simulink model "gm_uz_ssi_interface_2023a"  (R2023a)
settings: Solver=FixedStepDiscrete  StartTime=0.0  StopTime=0.0025  RelTol=1e-3
undefined symbols (not defined in the file or in its folder): binary_or_gray, bit_sum, delay_first_clk_on_off, f_ADC, f_clock, PLL, ssi_clk_divider, ssi_encoder_bit_width_multi_turn, ssi_encoder_bit_width_single_turn, ssi_encoder_number_of_status_bits, t_ADC, t_clock
libraries: hdlmdlgenlib x111, hdlsllib x62, simulink x27, simulink_extras x7
(part 1 of 4)
settings Model: Creator=micha  LastModifiedBy=micha
settings SolverCC: AlgebraicLoopSolver=TrustRegion
settings DataIOCC: LimitDataPoints=on  SaveOutput=off  SaveTime=off
settings OptimizationCC: BlockReduction=off  ConditionallyExecuteInputs=off  DefaultParameterBehavior=Inlined  LifeSpan=inf
settings DebuggingCC: AlgebraicLoopMsg=error  ArtificialAlgebraicLoopMsg=none  InheritedTsInSrcMsg=none  SingleTaskRateTransMsg=error  UnconnectedInputMsg=warning  UnconnectedOutputMsg=warning  UnconnectedLineMsg=warning  AllowSymbolicDim=off  StrictBusMsg=ErrorOnBusTreatedAsVector  SFUnexpectedBacktrackingDiag=warning  SFNoUnconditionalDefaultTransitionDiag=warning  SFExecutionAtInitializationDiag=none  ArithmeticOperatorsInVariantConditions=warning
settings HardwareCC: ProdBitPerPointer=32  ProdBitPerSizeT=32  ProdBitPerPtrDiffT=32  ProdLargestAtomicFloat=None  ProdIntDivRoundTo=Undefined  ProdEndianess=Unspecified  ProdWordSize=32  ProdHWDeviceType=ASIC/FPGA->ASIC/FPGA  ProdEqTarget=off
settings ModelReferenceCC: EnableRefExpFcnMdlSchedulingChecks=on
settings SFSimCC: SimUseLocalCustomCode=off  CustomCodeUndefinedFunction=UseInterfaceOnly
settings RTWCC: RTWUseLocalCustomCode=off  DLArmComputeVersion=19.05
settings CodeAppCC: StateflowObjectComments=on
settings GRTTargetCC: TargetLangStandard=C89/C90 (ANSI)
settings ConfigComp: CovScope=ReferencedModels  CovMetricSettings=dw  CovSaveCumulativeToWorkspaceVar=on  CovSaveSingleToWorkspaceVar=on  CovExternalEMLEnable=off  CovSFcnEnable=off

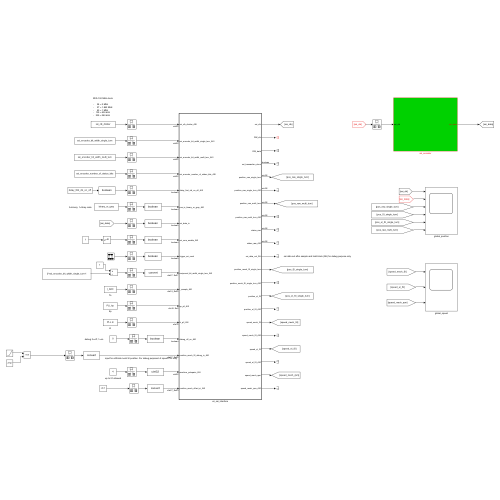
[thumbnail: Simulink's stored preview of the top-level diagram]
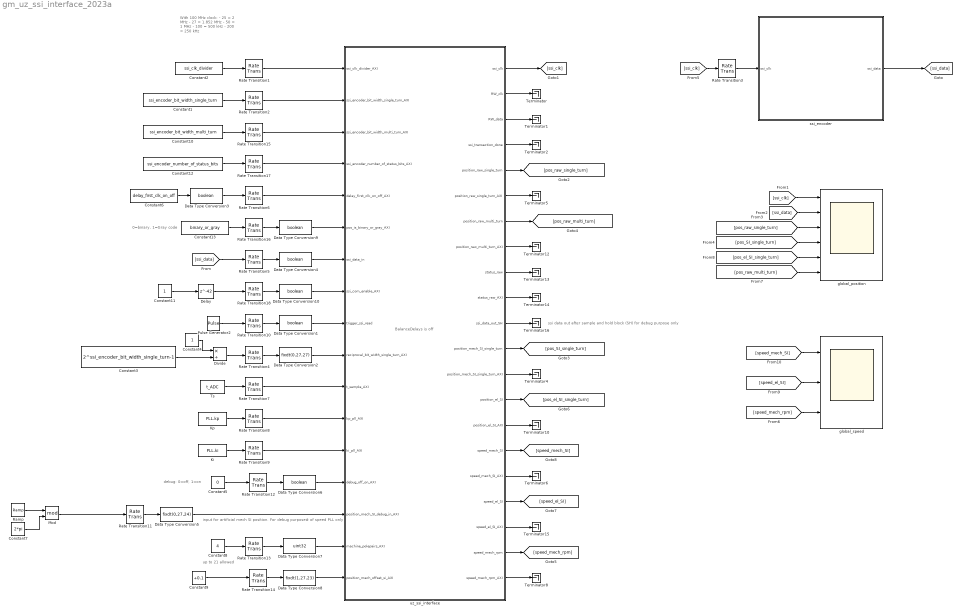
== system gm_uz_ssi_interface_2023a ==
  note: 0=binary, 1=Gray code
  note: With 100 MHz clock:
      |
      | -     25 = 2 MHz
      | -     27 = 1.852 MHz
      | -     50 = 1 MHz
      | -   100 = 500 kHz
      | -   200 = 250 kHz
  note: BalanceDelays is off
  note: debug: 0=off, 1=on
  note: up to 21 allowed
  note: ssi data out after sample and hold block (SH) for debug purpose only
  note: input for artificial mech SI position. For debug purpose# of speed PLL only
  Constant1 : Constant  Value=ssi_encoder_bit_width_single_turn  OutDataTypeStr=uint32  SampleTime=t_clock
  Constant10 : Constant  Value=ssi_encoder_bit_width_multi_turn  OutDataTypeStr=uint32  SampleTime=t_clock
  Constant11 : Constant  SampleTime=t_clock
  Constant12 : Constant  Value=ssi_encoder_number_of_status_bits  OutDataTypeStr=uint32  SampleTime=t_clock
  Constant13 : Constant  Value=binary_or_gray  OutDataTypeStr=uint32  SampleTime=t_clock
  Constant2 : Constant  Value=ssi_clk_divider  OutDataTypeStr=uint32  SampleTime=t_clock
  Constant3 : Constant  Value=2^ssi_encoder_bit_width_single_turn-1  OutDataTypeStr=double  SampleTime=t_clock
  Constant4 : Constant  SampleTime=t_clock
  Constant5 : Constant  Value=0  SampleTime=t_clock
  Constant6 : Constant  Value=delay_first_clk_on_off  OutDataTypeStr=uint32  SampleTime=t_clock
  Constant7 : Constant  Value=2*pi  SampleTime=t_clock
  Constant8 : Constant  Value=4  SampleTime=t_clock
  Constant9 : Constant  Value=+0.1  SampleTime=t_clock
  Data Type Conversion{1,3..4,6,9..10} (6 alike) : DataTypeConversion  OutDataTypeStr=boolean  SaturateOnIntegerOverflow=off  RndMeth=Floor
  Data Type Conversion2 : DataTypeConversion  OutDataTypeStr=fixdt(0,27,27)  SaturateOnIntegerOverflow=off  RndMeth=Floor
  Data Type Conversion5 : DataTypeConversion  OutDataTypeStr=fixdt(0,27,24)  SaturateOnIntegerOverflow=off  RndMeth=Floor
  Data Type Conversion7 : DataTypeConversion  OutDataTypeStr=uint32  SaturateOnIntegerOverflow=off  RndMeth=Floor
  Data Type Conversion8 : DataTypeConversion  OutDataTypeStr=fixdt(1,27,23)  SaturateOnIntegerOverflow=off  RndMeth=Floor
  Delay : Delay  DelayLength=42
  Divide : Product  Inputs=*/
  Ki : Constant  Value=PLL.ki  OutDataTypeStr=fixdt(0,18,0)  SampleTime=-1
  Kp : Constant  Value=PLL.kp  OutDataTypeStr=fixdt(0,18,5)  SampleTime=-1
  Mod : Math  Operator=mod
  Pulse Generator2 : DiscretePulseGenerator  Period=f_clock/f_ADC  PulseWidth=0.04*f_clock/f_ADC  PhaseDelay=250  SampleTime=t_clock
  Ramp : simulink/Sources/Ramp  slope=2*pi*100  start=7.5e-5  InitialOutput=0
  Rate Transition{1..18} (18 alike) : RateTransition  OutPortSampleTime=t_clock
  Terminator{,1..2,4..6,8,10,12..16} (13 alike) : Terminator
  Ts : Constant  Value=t_ADC  OutDataTypeStr=fixdt(0,18,24)  SampleTime=-1
  global_position : Scope  NumInputPorts=6
  global_speed : Scope  NumInputPorts=3
  ssi_encoder : Subsystem
  uz_ssi_interface : Subsystem  TreatAsAtomicUnit=on
  wires:
  [speed_el_SI] -> global_speed/2
  [speed_mech_SI] -> global_speed/1
  [pos_el_SI_single_turn] -> global_position/5
  [pos_raw_multi_turn] -> global_position/6
  [speed_mech_rpm] -> global_speed/3
  [ssi_clk] -> Rate Transition3/1
  Delay/1 -> Rate Transition18/1
  uz_ssi_interface/20(speed_mech_rpm) -> [speed_mech_rpm]
  uz_ssi_interface/11(ssi_data_out_SH) -> Terminator16/1
  uz_ssi_interface/12(position_mech_SI_single_turn) -> [pos_SI_single_turn]
  [pos_SI_single_turn] -> global_position/4
  [pos_raw_single_turn] -> global_position/3
  uz_ssi_interface/5(position_raw_single_turn) -> [pos_raw_single_turn]
  [ssi_data] -> global_position/2
  [ssi_clk] -> global_position/1
  uz_ssi_interface/18(speed_el_SI) -> [speed_el_SI]
  uz_ssi_interface/19(speed_el_SI_AXI) -> Terminator15/1
  uz_ssi_interface/10(status_raw_AXI) -> Terminator14/1
  uz_ssi_interface/9(status_raw) -> Terminator13/1
  uz_ssi_interface/8(position_raw_multi_turn_AXI) -> Terminator12/1
  uz_ssi_interface/7(position_raw_multi_turn) -> [pos_raw_multi_turn]
  Constant11/1 -> Delay/1
  Rate Transition18/1 -> Data Type Conversion10/1
  Data Type Conversion10/1 -> uz_ssi_interface/8(ssi_com_enable_AXI)
  Constant12/1 -> Rate Transition17/1
  Rate Transition17/1 -> uz_ssi_interface/4(ssi_encoder_number_of_status_bits_AXI)
  Data Type Conversion9/1 -> uz_ssi_interface/6(pos_is_binary_or_gray_AXI)
  Constant13/1 -> Rate Transition16/1
  Rate Transition16/1 -> Data Type Conversion9/1
  Constant10/1 -> Rate Transition15/1
  Rate Transition15/1 -> uz_ssi_interface/3(ssi_encoder_bit_width_multi_turn_AXI)
  uz_ssi_interface/15(position_el_SI_AXI) -> Terminator10/1
  uz_ssi_interface/14(position_el_SI) -> [pos_el_SI_single_turn]
  Data Type Conversion8/1 -> uz_ssi_interface/17(position_mech_offset_si_AXI)
  Constant9/1 -> Rate Transition14/1
  Rate Transition14/1 -> Data Type Conversion8/1
  Constant8/1 -> Rate Transition13/1
  Data Type Conversion7/1 -> uz_ssi_interface/16(machine_polepairs_AXI)
  Rate Transition13/1 -> Data Type Conversion7/1
  uz_ssi_interface/21(speed_mech_rpm_AXI) -> Terminator8/1
  Constant7/1 -> Mod/2
  Ramp/1 -> Mod/1
  Mod/1 -> Rate Transition11/1
  Constant5/1 -> Rate Transition12/1
  Rate Transition12/1 -> Data Type Conversion6/1
  Data Type Conversion6/1 -> uz_ssi_interface/14(debug_off_on_AXI)
  Data Type Conversion5/1 -> uz_ssi_interface/15(position_mech_SI_debug_in_AXI)
  Rate Transition11/1 -> Data Type Conversion5/1
  uz_ssi_interface/17(speed_mech_SI_AXI) -> Terminator6/1
  uz_ssi_interface/16(speed_mech_SI) -> [speed_mech_SI]
  Rate Transition9/1 -> uz_ssi_interface/13(ki_pll_AXI)
  Ki/1 -> Rate Transition9/1
  Rate Transition8/1 -> uz_ssi_interface/12(kp_pll_AXI)
  Kp/1 -> Rate Transition8/1
  Rate Transition7/1 -> uz_ssi_interface/11(t_sample_AXI)
  Ts/1 -> Rate Transition7/1
  uz_ssi_interface/13(position_mech_SI_single_turn_AXI) -> Terminator4/1
  Divide/1 -> Rate Transition4/1
  Constant4/1 -> Divide/1
  Data Type Conversion2/1 -> uz_ssi_interface/10(reciprocal_bit_width_single_turn_AXI)
  Rate Transition4/1 -> Data Type Conversion2/1
  Constant3/1 -> Divide/2
  Data Type Conversion4/1 -> uz_ssi_interface/7(ssi_data_in)
  Rate Transition5/1 -> Data Type Conversion4/1
  uz_ssi_interface/6(position_raw_single_turn_AXI) -> Terminator5/1
  Constant6/1 -> Data Type Conversion3/1
  Data Type Conversion3/1 -> Rate Transition6/1
  Rate Transition6/1 -> uz_ssi_interface/5(delay_first_clk_on_off_AXI)
  Data Type Conversion1/1 -> uz_ssi_interface/9(trigger_ssi_read)
  uz_ssi_interface/2(RW_clk) -> Terminator/1
  uz_ssi_interface/4(ssi_transaction_done) -> Terminator2/1
  uz_ssi_interface/3(RW_data) -> Terminator1/1
  uz_ssi_interface/1(ssi_clk) -> [ssi_clk]
  [ssi_data] -> Rate Transition5/1
  ssi_encoder/1(ssi_data) -> [ssi_data]
  Rate Transition3/1 -> ssi_encoder/1(ssi_clk)
  Rate Transition2/1 -> uz_ssi_interface/2(ssi_encoder_bit_width_single_turn_AXI)
  Constant1/1 -> Rate Transition2/1
  Rate Transition1/1 -> uz_ssi_interface/1(ssi_clk_divider_AXI)
  Constant2/1 -> Rate Transition1/1
  Pulse Generator2/1 -> Rate Transition10/1
  Rate Transition10/1 -> Data Type Conversion1/1

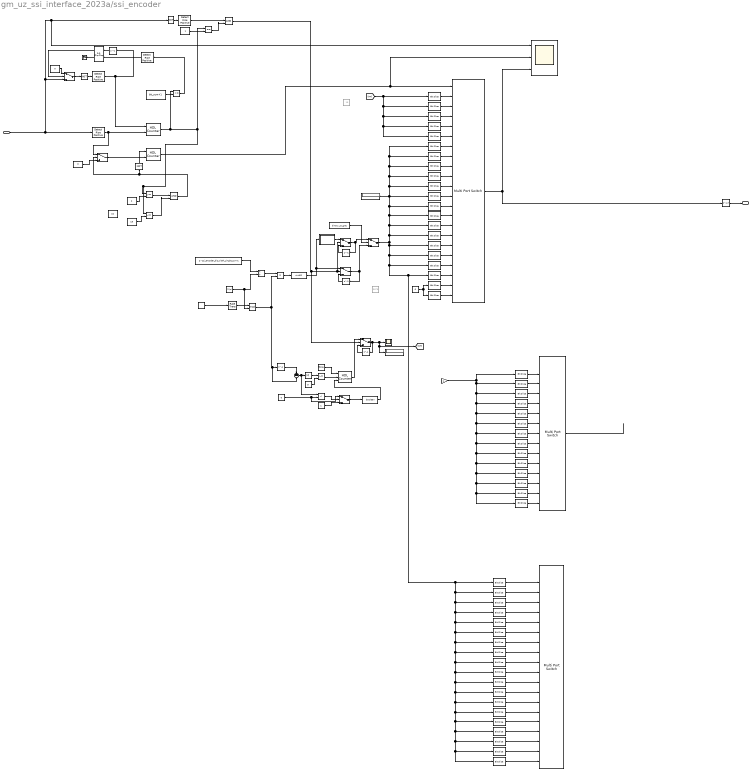
== system gm_uz_ssi_interface_2023a/ssi_encoder ==
  note: 19 bit single turn
  note: singleturn information
  note: Detect first falling edge of the clock
  note: 170 ns delay of the readhead
  note: multiturn information
  note: 14 bit single turn
  note: 5bit multiturn, 14bit single turn 2bit status
  ssi_clk : Inport
  AND : Logic  IconShape=distinctive  AllPortsSameDT=off  OutDataTypeStr=boolean
  AND1 : Logic  IconShape=distinctive  AllPortsSameDT=off  OutDataTypeStr=boolean
  Abs : Abs  SaturateOnIntegerOverflow=off
  Bit Slice{1,14,19,26,40} (5 alike) : hdlsllib/Logic and Bit Operations/Bit Slice  lidx=1  ridx=1
  Bit Slice10 : hdlsllib/Logic and Bit Operations/Bit Slice  lidx=5  ridx=5
  Bit Slice{11,16,23,37} (4 alike) : hdlsllib/Logic and Bit Operations/Bit Slice  lidx=4  ridx=4
  Bit Slice{12,17,24,38} (4 alike) : hdlsllib/Logic and Bit Operations/Bit Slice  lidx=3  ridx=3
  Bit Slice{13,18,25,39} (4 alike) : hdlsllib/Logic and Bit Operations/Bit Slice  lidx=2  ridx=2
  Bit Slice{15,20..21,27,41} (5 alike) : hdlsllib/Logic and Bit Operations/Bit Slice  lidx=0  ridx=0
  Bit Slice2 : hdlsllib/Logic and Bit Operations/Bit Slice  lidx=13  ridx=13
  Bit Slice22 : hdlsllib/Logic and Bit Operations/Bit Slice  lidx=5  ridx=5
  Bit Slice28 : hdlsllib/Logic and Bit Operations/Bit Slice  lidx=13  ridx=13
  Bit Slice29 : hdlsllib/Logic and Bit Operations/Bit Slice  lidx=12  ridx=12
  Bit Slice3 : hdlsllib/Logic and Bit Operations/Bit Slice  lidx=12  ridx=12
  Bit Slice30 : hdlsllib/Logic and Bit Operations/Bit Slice  lidx=11  ridx=11
  Bit Slice31 : hdlsllib/Logic and Bit Operations/Bit Slice  lidx=10  ridx=10
  Bit Slice32 : hdlsllib/Logic and Bit Operations/Bit Slice  lidx=9  ridx=9
  Bit Slice33 : hdlsllib/Logic and Bit Operations/Bit Slice  lidx=8  ridx=8
  Bit Slice34 : hdlsllib/Logic and Bit Operations/Bit Slice  lidx=7  ridx=7
  Bit Slice35 : hdlsllib/Logic and Bit Operations/Bit Slice  lidx=6  ridx=6
  Bit Slice36 : hdlsllib/Logic and Bit Operations/Bit Slice  lidx=5  ridx=5
  Bit Slice4 : hdlsllib/Logic and Bit Operations/Bit Slice  lidx=11  ridx=11
  Bit Slice42 : hdlsllib/Logic and Bit Operations/Bit Slice  lidx=13  ridx=13
  Bit Slice43 : hdlsllib/Logic and Bit Operations/Bit Slice  lidx=12  ridx=12
  Bit Slice44 : hdlsllib/Logic and Bit Operations/Bit Slice  lidx=11  ridx=11
  Bit Slice45 : hdlsllib/Logic and Bit Operations/Bit Slice  lidx=10  ridx=10
  Bit Slice46 : hdlsllib/Logic and Bit Operations/Bit Slice  lidx=9  ridx=9
  Bit Slice47 : hdlsllib/Logic and Bit Operations/Bit Slice  lidx=8  ridx=8
  Bit Slice48 : hdlsllib/Logic and Bit Operations/Bit Slice  lidx=7  ridx=7
  Bit Slice49 : hdlsllib/Logic and Bit Operations/Bit Slice  lidx=6  ridx=6
  Bit Slice5 : hdlsllib/Logic and Bit Operations/Bit Slice  lidx=10  ridx=10
  Bit Slice50 : hdlsllib/Logic and Bit Operations/Bit Slice  lidx=18  ridx=18
  Bit Slice51 : hdlsllib/Logic and Bit Operations/Bit Slice  lidx=17  ridx=17
  Bit Slice52 : hdlsllib/Logic and Bit Operations/Bit Slice  lidx=16  ridx=16
  Bit Slice53 : hdlsllib/Logic and Bit Operations/Bit Slice  lidx=15  ridx=15
  Bit Slice54 : hdlsllib/Logic and Bit Operations/Bit Slice  lidx=14  ridx=14
  Bit Slice6 : hdlsllib/Logic and Bit Operations/Bit Slice  lidx=9  ridx=9
  Bit Slice7 : hdlsllib/Logic and Bit Operations/Bit Slice  lidx=8  ridx=8
  Bit Slice8 : hdlsllib/Logic and Bit Operations/Bit Slice  lidx=7  ridx=7
  Bit Slice9 : hdlsllib/Logic and Bit Operations/Bit Slice  lidx=6  ridx=6
  Constant : Constant  Value=bit_sum+1  SampleTime=t_clock
  Constant1 : Constant  Value=0  SampleTime=t_clock
  Constant10 : Constant  Value=false  SampleTime=t_clock
  Constant11 : Constant  Value=0  SampleTime=t_clock
  Constant12 : Constant  SampleTime=t_clock
  Constant13 : Constant  Value=0  OutDataTypeStr=uint32  SampleTime=t_clock
  Constant14 : Constant  Commented=on  Value=19  OutDataTypeStr=uint32  SampleTime=t_clock
  Constant15 : Constant  Value=binary_or_gray  SampleTime=t_clock
  Constant16 : Constant  Value=15  SampleTime=t_clock
  Constant2 : Constant  SampleTime=t_clock
  Constant3 : Constant  Value=0  OutDataTypeStr=boolean  SampleTime=t_clock
  Constant4 : Constant  Value=5  SampleTime=t_clock
  Constant5 : Constant  Value=2  SampleTime=t_clock
  Constant6 : Constant  Commented=on  Value=3875  OutDataTypeStr=uint32  SampleTime=t_clock
  Constant7 : Constant  Value=2*pi  SampleTime=t_clock
  Constant8 : Constant  Value=22  SampleTime=t_clock
  Constant9 : Constant  Value=2^ssi_encoder_bit_width_single_turn-1  SampleTime=t_clock
  Data Type Conversion : DataTypeConversion  OutDataTypeStr=uint32  SaturateOnIntegerOverflow=off  RndMeth=Floor
  Data Type Conversion1 : DataTypeConversion  OutDataTypeStr=boolean  SaturateOnIntegerOverflow=off  RndMeth=Floor
  Delay : Delay  DelayLength=1
  Delay1 : Delay  DelayLength=17  SampleTime=t_clock
  Delay2 : Delay  DelayLength=1  SampleTime=t_clock
  Delay3 : Delay  DelayLength=1
  Delay4 : Delay  DelayLength=1  InitialCondition=19  SampleTime=t_clock
  Delay5 : Delay  DelayLength=1  SampleTime=t_clock
  Detect Rise Positive{,1..3} (4 alike) : simulink/Logic and Bit Operations/Detect Rise Positive  vinit=0  OutDataTypeStr=boolean
  Display : Display
  Display1 : Display
  Divide : Product  Inputs=*/
  Gain : Gain
  HDL Counter : hdlsllib/Sources/HDL Counter  CountType=Count limited  CountInit=0  CountStep=1  CountMax=bit_sum+1  CountFromType=Initial value  CountFrom=0  CountResetPort=on  CountLoadPort=off  CountEnbPort=on  CountDirPort=off  CountHitOutputPort=off  CountDataType=Unsigned  CountWordLen=8  CountFracLen=0  CountSampTime=t_clock
  HDL Counter1 : hdlsllib/Sources/HDL Counter  CountType=Count limited  CountInit=0  CountStep=1  CountMax=bit_sum+1  CountFromType=Initial value  CountFrom=0  CountResetPort=on  CountLoadPort=off  CountEnbPort=on  CountDirPort=off  CountHitOutputPort=off  CountDataType=Unsigned  CountWordLen=8  CountFracLen=0  CountSampTime=t_clock
  HDL Counter2 : hdlsllib/Sources/HDL Counter  CountType=Count limited  CountInit=19  CountStep=1  CountMax=ssi_encoder_bit_width_multi_turn  CountFromType=Initial value  CountFrom=19  CountResetPort=on  CountLoadPort=off  CountEnbPort=on  CountDirPort=on  CountHitOutputPort=off  CountDataType=Unsigned  CountWordLen=5  CountFracLen=0  CountSampTime=t_clock
  Index Vector : MultiPortSwitch  DataPortOrder=Zero-based contiguous  Inputs=21  zeroidx=on  SaturateOnIntegerOverflow=off  InputSameDT=off
  Index Vector1 : MultiPortSwitch  DataPortOrder=Zero-based contiguous  Inputs=14  zeroidx=on  SaturateOnIntegerOverflow=off  InputSameDT=off
  Index Vector2 : MultiPortSwitch  DataPortOrder=Zero-based contiguous  Inputs=19  zeroidx=on  SaturateOnIntegerOverflow=off  InputSameDT=off
  MATLAB Function : MATLAB Function  TreatAsAtomicUnit=on
  Mod : Math  Operator=mod
  NOT : Logic  Operator=NOT  IconShape=distinctive  AllPortsSameDT=off  OutDataTypeStr=boolean
  NOT1 : Logic  Operator=NOT  IconShape=distinctive  AllPortsSameDT=off  OutDataTypeStr=boolean
  NOT2 : Logic  Operator=NOT  IconShape=distinctive  AllPortsSameDT=off  OutDataTypeStr=boolean
  Product : Product
  Ramp : simulink/Sources/Ramp  slope=-2*pi*50  start=7.5e-5  InitialOutput=0
  Rate Transition : RateTransition  OutPortSampleTime=t_clock
  Relational Operator : RelationalOperator  OutDataTypeStr=boolean  RndMeth=Simplest  InputSameDT=off
  Relational Operator1 : RelationalOperator  OutDataTypeStr=boolean  RndMeth=Simplest  InputSameDT=off
  Relational Operator2 : RelationalOperator  Operator===  OutDataTypeStr=boolean  RndMeth=Simplest  InputSameDT=off
  Relational Operator3 : RelationalOperator  Operator=<=  OutDataTypeStr=boolean  RndMeth=Simplest  InputSameDT=off
  Relational Operator4 : RelationalOperator  OutDataTypeStr=boolean  RndMeth=Simplest  InputSameDT=off
  Relational Operator5 : RelationalOperator  Operator=<  OutDataTypeStr=boolean  RndMeth=Simplest  InputSameDT=off
  S-R Flip-Flop : simulink_extras/Flip Flops/S-R Flip-Flop  initial_condition=0
  Scope : Scope  NumInputPorts=3
  Scope1 : Scope
  Sum : Sum  Inputs=+-
  Switch{,1..6} (7 alike) : Switch  Criteria=u2 > Threshold  SaturateOnIntegerOverflow=off  InputSameDT=off
  Terminator : Terminator
  ssi_data : Outport
  wires:
  Gain/1 -> Bit Slice29/1, Bit Slice30/1, Bit Slice31/1, Bit Slice32/1, Bit Slice33/1, Bit Slice34/1, Bit Slice35/1, Bit Slice22/1, Bit Slice23/1, Bit Slice24/1, Bit Slice25/1, Bit Slice26/1, Bit Slice27/1, Bit Slice28/1
  Index Vector/1 -> Delay1/1, Scope/3
  Switch5/1 -> Bit Slice11/1, Bit Slice10/1, Bit Slice9/1, Bit Slice8/1, Bit Slice7/1, Bit Slice3/1, Bit Slice2/1, Bit Slice4/1, Bit Slice5/1, Bit Slice6/1, Display/1, Bit Slice12/1, Bit Slice13/1, Bit Slice14/1, Bit Slice15/1, Bit Slice50/1, Bit Slice51/1, Bit Slice52/1, Bit Slice53/1, Bit Slice54/1, Bit Slice42/1, Bit Slice43/1, Bit Slice44/1, Bit Slice45/1, Bit Slice46/1, Bit Slice47/1, Bit Slice48/1, Bit Slice49/1, Bit Slice36/1, Bit Slice41/1, Bit Slice40/1, Bit Slice39/1, Bit Slice38/1, Bit Slice37/1
  Bit Slice51/1 -> Index Vector2/3
  Bit Slice54/1 -> Index Vector2/6
  Bit Slice50/1 -> Index Vector2/2
  Bit Slice53/1 -> Index Vector2/5
  Bit Slice52/1 -> Index Vector2/4
  Bit Slice39/1 -> Index Vector2/18
  Bit Slice49/1 -> Index Vector2/14
  Bit Slice43/1 -> Index Vector2/8
  Bit Slice48/1 -> Index Vector2/13
  Bit Slice46/1 -> Index Vector2/11
  Bit Slice45/1 -> Index Vector2/10
  Bit Slice38/1 -> Index Vector2/17
  Bit Slice42/1 -> Index Vector2/7
  Bit Slice41/1 -> Index Vector2/20
  Bit Slice44/1 -> Index Vector2/9
  Bit Slice36/1 -> Index Vector2/15
  Bit Slice40/1 -> Index Vector2/19
  Bit Slice37/1 -> Index Vector2/16
  Bit Slice47/1 -> Index Vector2/12
  Index Vector1/1 -> ?
  Bit Slice24/1 -> Index Vector1/12
  Bit Slice25/1 -> Index Vector1/13
  Bit Slice32/1 -> Index Vector1/6
  Bit Slice30/1 -> Index Vector1/4
  Bit Slice35/1 -> Index Vector1/9
  Bit Slice27/1 -> Index Vector1/15
  Bit Slice31/1 -> Index Vector1/5
  Bit Slice23/1 -> Index Vector1/11
  Bit Slice34/1 -> Index Vector1/8
  Bit Slice28/1 -> Index Vector1/2
  Bit Slice22/1 -> Index Vector1/10
  Bit Slice26/1 -> Index Vector1/14
  Bit Slice33/1 -> Index Vector1/7
  Bit Slice29/1 -> Index Vector1/3
  Delay5/1 -> Switch6/3
  Switch6/1 -> Switch5/1, Delay5/1
  MATLAB Function/1(y) -> Switch6/1
  Switch1/1 -> Switch5/3, Delay2/1
  Constant15/1 -> Switch5/2
  Data Type Conversion1/1 -> HDL Counter2/3
  Constant13/1 -> Bit Slice21/1, Bit Slice1/1
  Bit Slice21/1 -> Index Vector/22
  Bit Slice1/1 -> Index Vector/21
  Bit Slice15/1 -> Index Vector/20
  Bit Slice14/1 -> Index Vector/19
  Bit Slice13/1 -> Index Vector/18
  Bit Slice12/1 -> Index Vector/17
  Bit Slice11/1 -> Index Vector/16
  Bit Slice10/1 -> Index Vector/15
  Bit Slice9/1 -> Index Vector/14
  Bit Slice8/1 -> Index Vector/13
  Bit Slice7/1 -> Index Vector/12
  Bit Slice6/1 -> Index Vector/11
  Bit Slice5/1 -> Index Vector/10
  Bit Slice4/1 -> Index Vector/9
  Bit Slice3/1 -> Index Vector/8
  Bit Slice2/1 -> Index Vector/7
  Bit Slice20/1 -> Index Vector/6
  Bit Slice19/1 -> Index Vector/5
  Bit Slice18/1 -> Index Vector/4
  Bit Slice17/1 -> Index Vector/3
  Bit Slice16/1 -> Index Vector/2
  [MT] -> Bit Slice16/1, Bit Slice20/1, Bit Slice19/1, Bit Slice18/1, Bit Slice17/1
  Constant12/1 -> Switch4/3
  Switch4/1 -> Data Type Conversion1/1
  Relational Operator5/1 -> Switch4/2
  Constant11/1 -> Relational Operator5/2, Switch4/1
  Constant10/1 -> HDL Counter2/1
  Switch2/1 -> Delay4/1, Scope1/1, Display1/1, [MT]
  Delay4/1 -> Switch2/3
  HDL Counter2/1 -> Switch2/1
  Relational Operator4/1 -> HDL Counter2/2
  Constant4/1 -> Relational Operator4/2
  Abs/1 -> Relational Operator4/1
  Sum/1 -> Abs/1, Relational Operator5/1
  Mod/1 -> Product/2, Delay3/1, Sum/2
  Delay3/1 -> Sum/1
  Delay1/1 -> ssi_data/1
  HDL Counter1/1 -> Index Vector/1, Scope/2
  Constant3/1 -> Switch3/3
  AND/1 -> Switch1/2, Switch6/2, Switch2/2
  Data Type Conversion/1 -> MATLAB Function/1(u), Switch1/1
  Delay2/1 -> Switch1/3
  Rate Transition/1 -> Mod/1
  Product/1 -> Data Type Conversion/1
  Constant7/1 -> Divide/2, Mod/2
  Divide/1 -> Product/1
  Constant9/1 -> Divide/1
  Ramp/1 -> Rate Transition/1
  NOT2/1 -> HDL Counter1/1
  Switch3/1 -> HDL Counter1/2
  Constant16/1 -> Relational Operator3/2
  Relational Operator3/1 -> AND1/2
  Constant5/1 -> Relational Operator1/2
  AND1/1 -> Switch3/2, NOT2/1
  Relational Operator1/1 -> AND1/1
  ssi_clk/1 -> Detect Rise Positive1/1, Switch/3, NOT1/1, Scope/1
  Constant1/1 -> Switch/1
  S-R Flip-Flop/2 -> Terminator/1
  HDL Counter/1 -> Relational Operator/1, Relational Operator2/1, Relational Operator1/1, Relational Operator3/1
  Detect Rise Positive1/1 -> Switch3/1, HDL Counter/2
  Detect Rise Positive3/1 -> AND/1
  NOT1/1 -> Detect Rise Positive3/1
  Constant2/1 -> Relational Operator2/2
  Relational Operator2/1 -> AND/2
  Detect Rise Positive/1 -> Delay/1, HDL Counter/1
  Detect Rise Positive2/1 -> S-R Flip-Flop/2
  Relational Operator/1 -> Detect Rise Positive2/1
  Delay/1 -> S-R Flip-Flop/1
  S-R Flip-Flop/1 -> Switch/2
  Switch/1 -> NOT/1
  Constant/1 -> Relational Operator/2
  NOT/1 -> Detect Rise Positive/1

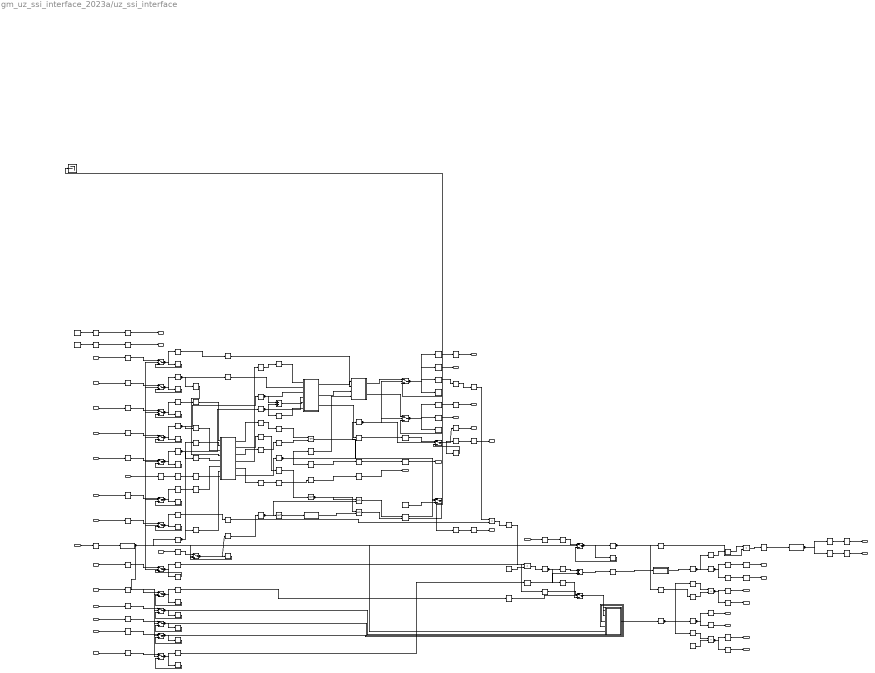
== system gm_uz_ssi_interface_2023a/uz_ssi_interface ==
  note: slice raw data and decode position
  note: mech speed SI to el speed SI
  note: encoder offset
  note: electrical position
  note: mech speed SI to mech speed RPM
  note: SI mech position to mech speed SI
  note: Acquisition of raw position data from the SSI absolute encoder
  note: Processing of raw position data
  note: raw mech position to SI mech position
  note: pull clk high when disabled
  note: enable logic for clock: turns on and off clk only between transmissions
  ssi_clk_divider_AXI : Inport  OutDataTypeStr=uint32  PortDimensions=1  SampleTime=1e-08
  ssi_encoder_bit_width_single_turn_AXI : Inport  Port=2  OutDataTypeStr=uint32  PortDimensions=1  SampleTime=1e-08
  ssi_encoder_bit_width_multi_turn_AXI : Inport  Port=3  OutDataTypeStr=uint32  PortDimensions=1  SampleTime=1e-08
  ssi_encoder_number_of_status_bits_AXI : Inport  Port=4  OutDataTypeStr=uint32  PortDimensions=1  SampleTime=1e-08
  delay_first_clk_on_off_AXI : Inport  Port=5  OutDataTypeStr=boolean  PortDimensions=1  SampleTime=1e-08
  pos_is_binary_or_gray_AXI : Inport  Port=6  OutDataTypeStr=boolean  PortDimensions=1  SampleTime=1e-08
  ssi_data_in : Inport  Port=7  OutDataTypeStr=boolean  PortDimensions=1  SampleTime=1e-08
  ssi_com_enable_AXI : Inport  Port=8  OutDataTypeStr=boolean  PortDimensions=1  SampleTime=1e-08
  trigger_ssi_read : Inport  Port=9  OutDataTypeStr=boolean  PortDimensions=1  SampleTime=1e-08
  reciprocal_bit_width_single_turn_AXI : Inport  Port=10  OutDataTypeStr=fixdt(0, 27, 27)  PortDimensions=1  SampleTime=1e-08
  t_sample_AXI : Inport  Port=11  OutDataTypeStr=fixdt(0, 18, 24)  PortDimensions=1  SampleTime=1e-08
  kp_pll_AXI : Inport  Port=12  OutDataTypeStr=fixdt(0, 18, 5)  PortDimensions=1  SampleTime=1e-08
  ki_pll_AXI : Inport  Port=13  OutDataTypeStr=fixdt(0, 18, 0)  PortDimensions=1  SampleTime=1e-08
  debug_off_on_AXI : Inport  Port=14  OutDataTypeStr=boolean  PortDimensions=1  SampleTime=1e-08
  position_mech_SI_debug_in_AXI : Inport  Port=15  OutDataTypeStr=fixdt(0, 27, 24)  PortDimensions=1  SampleTime=1e-08
  machine_polepairs_AXI : Inport  Port=16  OutDataTypeStr=uint32  PortDimensions=1  SampleTime=1e-08
  position_mech_offset_si_AXI : Inport  Port=17  OutDataTypeStr=fixdt(1, 27, 23)  PortDimensions=1  SampleTime=1e-08
  AND : Logic  AllPortsSameDT=off  OutDataTypeStr=boolean  SampleTime=1e-08
  AND1 : Logic  AllPortsSameDT=off  OutDataTypeStr=boolean  SampleTime=1e-08
  Constant : Constant  Value=6.283172607421875  OutDataTypeStr=fixdt(0, 18, 15)  SampleTime=1e-08
  Constant1 : Constant  OutDataTypeStr=boolean  SampleTime=1e-08
  Constant3 : Constant  Value=0  OutDataTypeStr=boolean  SampleTime=1e-08
  Constant4 : Constant  Value=9.54931640625  OutDataTypeStr=fixdt(0, 18, 14)  SampleTime=1e-08
  Constant5 : Constant  OutDataTypeStr=boolean  SampleTime=1e-08
  Data Type Conversion : DataTypeConversion  OutDataTypeStr=uint8  SampleTime=1e-08  SaturateOnIntegerOverflow=off  RndMeth=Floor
  Data Type Conversion1 : DataTypeConversion  OutDataTypeStr=int32  SampleTime=1e-08  SaturateOnIntegerOverflow=off  RndMeth=Floor
  Delay{,4,7..8,10..11,15..20,22,24,26..27,29,33..34,37,39..43,46,50..52,54..57,127,129} (35 alike) : Delay  DelayLength=double(1)  InitialCondition=0  SampleTime=1e-08
  Delay1 : Delay  DelayLength=double(1)  InitialCondition=14  SampleTime=1e-08
  Delay14 : Delay  DelayLength=double(1)  InitialCondition=1  SampleTime=1e-08
  Delay{2..3,6,9,21,23,25,28,30,32,36,38,45,47,49,53,64} (17 alike) : Delay  DelayLength=double(2)  InitialCondition=0  SampleTime=1e-08
  Delay31 : Delay  DelayLength=double(1)  InitialCondition=25  SampleTime=1e-08
  Delay35 : Delay  DelayLength=double(1)  InitialCondition=1  SampleTime=1e-08
  Delay44 : Delay  DelayLength=double(1)  InitialCondition=5  SampleTime=1e-08
  Delay48 : Delay  DelayLength=double(1)  InitialCondition=2  SampleTime=1e-08
  Detect Rise Positive : simulink/Logic and Bit Operations/Detect Rise Positive  vinit=0  OutDataTypeStr=boolean
  Detect Rise Positive1 : simulink/Logic and Bit Operations/Detect Rise Positive  vinit=0  OutDataTypeStr=boolean
  From{,1..8,11..25,27..32,35..40} (36 alike) : hdlmdlgenlib/Buffer
  Goto{,1..24} (25 alike) : hdlmdlgenlib/Buffer
  Gray_code_to_binary : Subsystem
  NOT : Logic  Operator=NOT  Inputs=1  AllPortsSameDT=off  OutDataTypeStr=boolean  SampleTime=1e-08
  NOT1 : Logic  Operator=NOT  Inputs=1  AllPortsSameDT=off  OutDataTypeStr=boolean  SampleTime=1e-08
  OR : Logic  Operator=OR  AllPortsSameDT=off  OutDataTypeStr=boolean  SampleTime=1e-08
  Product : Product  Inputs=**  OutDataTypeStr=fixdt(0, 27, 24)  SampleTime=1e-08
  Product1 : Product  Inputs=**  OutDataTypeStr=fixdt(1, 27, 12)  SampleTime=1e-08
  Product2 : Product  Inputs=**  OutDataTypeStr=fixdt(1, 27, 12)  SampleTime=1e-08
  Product4 : Product  Inputs=**  OutDataTypeStr=fixdt(0, 27, 20)  SampleTime=1e-08
  Product7 : Product  Inputs=**  OutDataTypeStr=fixdt(0, 27, 24)  SampleTime=1e-08
  S-R Flip-Flop1 : simulink_extras/Flip Flops/S-R Flip-Flop  initial_condition=0
  S-R Flip-Flop1_inst_term1 : Terminator
  Sum1 : Sum  AccumDataTypeStr=fixdt(1, 29, 24)  OutDataTypeStr=fixdt(1, 27, 23)  SampleTime=1e-08
  Sum2 : Sum  AccumDataTypeStr=fixdt(0, 33, 0)  OutDataTypeStr=int32  SampleTime=1e-08
  Switch{1,6,13,15..16,19,31} (7 alike) : Switch  Criteria=u2 > Threshold  Threshold=double(0)  OutDataTypeStr=uint32  SampleTime=1e-08  SaturateOnIntegerOverflow=off  InputSameDT=off
  Switch10 : Switch  Criteria=u2 > Threshold  Threshold=double(0)  OutDataTypeStr=fixdt(0, 27, 24)  SampleTime=1e-08  SaturateOnIntegerOverflow=off  InputSameDT=off
  Switch11 : Switch  Criteria=u2 > Threshold  Threshold=double(0)  OutDataTypeStr=uint8  SampleTime=1e-08  SaturateOnIntegerOverflow=off  InputSameDT=off
  Switch12 : Switch  Criteria=u2 > Threshold  Threshold=double(0)  OutDataTypeStr=fixdt(1, 27, 23)  SampleTime=1e-08  SaturateOnIntegerOverflow=off  InputSameDT=off
  Switch{5,8,14,17..18} (5 alike) : Switch  Criteria=u2 > Threshold  Threshold=double(0)  OutDataTypeStr=boolean  SampleTime=1e-08  SaturateOnIntegerOverflow=off  InputSameDT=off
  Switch2 : Switch  Criteria=u2 > Threshold  Threshold=double(0)  OutDataTypeStr=fixdt(0, 27, 27)  SampleTime=1e-08  SaturateOnIntegerOverflow=off  InputSameDT=off
  Switch3 : Switch  Criteria=u2 > Threshold  Threshold=double(0)  OutDataTypeStr=fixdt(0, 18, 24)  SampleTime=1e-08  SaturateOnIntegerOverflow=off  InputSameDT=off
  Switch4 : Switch  Criteria=u2 > Threshold  Threshold=double(0)  OutDataTypeStr=fixdt(0, 18, 5)  SampleTime=1e-08  SaturateOnIntegerOverflow=off  InputSameDT=off
  Switch7 : Switch  Criteria=u2 > Threshold  Threshold=double(0)  OutDataTypeStr=fixdt(0, 18, 0)  SampleTime=1e-08  SaturateOnIntegerOverflow=off  InputSameDT=off
  Switch9 : Switch  Criteria=u2 > Threshold  Threshold=double(0)  OutDataTypeStr=fixdt(0, 27, 24)  SampleTime=1e-08  SaturateOnIntegerOverflow=off  InputSameDT=off
  delayMatch{,1..15} (16 alike) : Delay  DelayLength=double(1)  InitialCondition=0  SampleTime=1e-08
  position_to_speed_pll : Subsystem
  slice_position_and_status : Subsystem
  ssi_communication : Subsystem
  wrap_2pi : Subsystem
  wrap_2pi_after_offset : Subsystem
  ssi_clk : Outport  SampleTime=1e-08
  RW_clk : Outport  Port=2  SampleTime=1e-08
  RW_data : Outport  Port=3  SampleTime=1e-08
  ssi_transaction_done : Outport  Port=4  OutDataTypeStr=boolean  SampleTime=1e-08  LockScale=on
  position_raw_single_turn : Outport  Port=5  OutDataTypeStr=uint32  SampleTime=1e-08  LockScale=on
  position_raw_single_turn_AXI : Outport  Port=6  OutDataTypeStr=uint32  SampleTime=1e-08  LockScale=on
  position_raw_multi_turn : Outport  Port=7  OutDataTypeStr=uint32  SampleTime=1e-08  LockScale=on
  position_raw_multi_turn_AXI : Outport  Port=8  OutDataTypeStr=uint32  SampleTime=1e-08  LockScale=on
  status_raw : Outport  Port=9  OutDataTypeStr=uint32  SampleTime=1e-08  LockScale=on
  status_raw_AXI : Outport  Port=10  OutDataTypeStr=uint32  SampleTime=1e-08  LockScale=on
  ssi_data_out_SH : Outport  Port=11  SampleTime=1e-08
  position_mech_SI_single_turn : Outport  Port=12  SampleTime=1e-08
  position_mech_SI_single_turn_AXI : Outport  Port=13  SampleTime=1e-08
  position_el_SI : Outport  Port=14  SampleTime=1e-08
  position_el_SI_AXI : Outport  Port=15  SampleTime=1e-08
  speed_mech_SI : Outport  Port=16  SampleTime=1e-08
  speed_mech_SI_AXI : Outport  Port=17  SampleTime=1e-08
  speed_el_SI : Outport  Port=18  SampleTime=1e-08
  speed_el_SI_AXI : Outport  Port=19  SampleTime=1e-08
  speed_mech_rpm : Outport  Port=20  SampleTime=1e-08
  speed_mech_rpm_AXI : Outport  Port=21  SampleTime=1e-08
  wires:
  ssi_clk_divider_AXI/1 -> Delay64/1
  ssi_encoder_bit_width_single_turn_AXI/1 -> Delay2/1
  ssi_encoder_bit_width_multi_turn_AXI/1 -> Delay45/1
  ssi_encoder_number_of_status_bits_AXI/1 -> Delay49/1
  delay_first_clk_on_off_AXI/1 -> Delay6/1
  pos_is_binary_or_gray_AXI/1 -> Delay47/1
  ssi_data_in/1 -> Delay3/1
  ssi_com_enable_AXI/1 -> Delay53/1
  trigger_ssi_read/1 -> Delay32/1
  reciprocal_bit_width_single_turn_AXI/1 -> Delay9/1
  t_sample_AXI/1 -> Delay21/1
  kp_pll_AXI/1 -> Delay23/1
  ki_pll_AXI/1 -> Delay25/1
  debug_off_on_AXI/1 -> Delay28/1
  position_mech_SI_debug_in_AXI/1 -> Delay30/1
  machine_polepairs_AXI/1 -> Delay36/1
  position_mech_offset_si_AXI/1 -> Delay38/1
  AND/1 -> S-R Flip-Flop1/1
  AND1/1 -> S-R Flip-Flop1/2
  Constant/1 -> Product7/2
  Constant1/1 -> Delay4/1
  Constant3/1 -> Delay7/1
  Constant4/1 -> Product1/2
  Constant5/1 -> Switch17/3
  Data Type Conversion/1 -> Switch11/1
  Data Type Conversion1/1 -> slice_position_and_status/6(shift_val_st)
  Delay/1 -> Product/1
  delayMatch12/1 -> position_mech_SI_single_turn/1
  delayMatch13/1 -> position_mech_SI_single_turn_AXI/1
  delayMatch1/1 -> ssi_clk/1
  delayMatch4/1 -> ssi_transaction_done/1
  delayMatch6/1 -> position_raw_single_turn_AXI/1
  delayMatch11/1 -> ssi_data_out_SH/1
  Delay18/1 -> speed_mech_SI_AXI/1
  Delay19/1 -> speed_mech_SI/1
  Delay2/1 -> Switch1/1
  Delay21/1 -> Switch3/1
  Delay23/1 -> Switch4/1
  Delay25/1 -> Switch7/1
  Delay26/1 -> Product7/1
  Delay28/1 -> Switch8/1
  Delay3/1 -> Goto3/1
  Delay30/1 -> Switch10/1
  Delay32/1 -> Detect Rise Positive1/1
  Delay33/1 -> speed_mech_rpm/1
  Delay34/1 -> speed_mech_rpm_AXI/1
  Delay36/1 -> Data Type Conversion/1
  Delay38/1 -> Switch12/1
  Delay39/1 -> Product4/1
  delayMatch2/1 -> RW_clk/1
  delayMatch14/1 -> position_el_SI/1
  Delay41/1 -> wrap_2pi_after_offset/1(input)
  delayMatch15/1 -> position_el_SI_AXI/1
  Delay43/1 -> wrap_2pi/1(input)
  Delay45/1 -> Switch13/1
  Delay47/1 -> Switch14/1
  Delay49/1 -> Switch15/1
  delayMatch8/1 -> position_raw_multi_turn_AXI/1
  Delay53/1 -> Switch18/1
  delayMatch10/1 -> status_raw_AXI/1
  Delay56/1 -> speed_el_SI/1
  Delay57/1 -> speed_el_SI_AXI/1
  Delay6/1 -> Switch5/1
  Delay64/1 -> Switch31/1
  delayMatch3/1 -> RW_data/1
  Delay9/1 -> Switch2/1
  Detect Rise Positive/1 -> AND1/2
  Detect Rise Positive1/1 -> Goto22/1, position_to_speed_pll/5(Trigger), Switch31/2, Switch1/2, Switch13/2, Switch15/2, Switch5/2, Switch11/2, Switch18/2, Switch14/2, Switch2/2, Switch12/2, Switch10/2, Switch8/2, Switch3/2, Switch4/2, Switch7/2
  From/1 -> Delay129/1
  From1/1 -> ssi_communication/6(delay_first_clk_on_off)
  From11/1 -> Switch9/2
  From12/1 -> Switch9/3
  From13/1 -> Switch9/1
  From14/1 -> Product1/1
  From15/1 -> Switch6/2, Switch16/2, Switch19/2
  From16/1 -> Product4/2
  From17/1 -> Gray_code_to_binary/2(pos_is_binary_or_gray)
  From18/1 -> slice_position_and_status/1(data)
  From19/1 -> Sum1/1
  From2/1 -> Delay/1
  From20/1 -> Sum1/2
  From21/1 -> Delay11/1, Delay10/1
  From22/1 -> Delay39/1
  From23/1 -> ssi_communication/3(In3)
  From24/1 -> ssi_communication/4(In4)
  From25/1 -> ssi_communication/5(In5)
  From27/1 -> NOT1/1, AND/2
  From28/1 -> NOT/1
  From29/1 -> Delay17/1
  From3/1 -> Delay19/1, Delay18/1
  From30/1 -> Switch19/1
  From31/1 -> Product2/1
  delayMatch/1 -> Product2/2
  From35/1 -> slice_position_and_status/2(bit_width_mt)
  From36/1 -> Sum2/1, slice_position_and_status/3(bit_width_st)
  From37/1 -> Sum2/2, Data Type Conversion1/1, slice_position_and_status/4(bit_width_status)
  From38/1 -> ssi_communication/2(ssi_clk_reset)
  From39/1 -> ssi_communication/7(trigger_ssi)
  From4/1 -> ssi_communication/1(ssi_clk_divider)
  From40/1 -> OR/2
  From5/1 -> OR/1
  From6/1 -> Product/2
  From7/1 -> ssi_communication/8(ssi_data_in)
  From8/1 -> Gray_code_to_binary/4(trigger)
  Gray_code_to_binary/1(ssi_pos_single_turn_binary) -> Switch6/1
  Gray_code_to_binary/2(ssi_pos_multi_turn_binary) -> Switch16/1
  NOT/1 -> AND1/1, AND/1
  NOT1/1 -> Detect Rise Positive/1
  OR/1 -> Switch17/1
  Product/1 -> Delay26/1
  Product1/1 -> Delay34/1, Delay33/1
  Product2/1 -> Delay57/1, Delay56/1
  Product4/1 -> Delay43/1
  Product7/1 -> Goto2/1
  S-R Flip-Flop1/1 -> Switch17/2
  S-R Flip-Flop1/2 -> S-R Flip-Flop1_inst_term1/1
  Sum1/1 -> Delay41/1
  Sum2/1 -> slice_position_and_status/5(shift_val_mt)
  Switch1/1 -> Goto/1, Delay1/1
  Switch10/1 -> Goto10/1, Delay29/1
  Switch11/1 -> Goto11/1, Delay35/1
  Switch12/1 -> Goto13/1, Delay37/1
  Switch13/1 -> Goto15/1, Delay44/1
  Switch14/1 -> Goto16/1, Delay46/1
  Switch15/1 -> Goto9/1, Delay48/1
  delayMatch7/1 -> position_raw_multi_turn/1
  Switch17/1 -> Delay127/1
  Switch18/1 -> Goto18/1, Delay52/1
  delayMatch9/1 -> status_raw/1
  Switch2/1 -> Goto5/1, Delay8/1
  Switch3/1 -> position_to_speed_pll/2(t_sample), Delay20/1
  Switch31/1 -> Goto7/1, Delay31/1
  Switch4/1 -> position_to_speed_pll/3(kp_pll), Delay22/1
  Switch5/1 -> Goto1/1, Delay14/1
  delayMatch5/1 -> position_raw_single_turn/1
  Switch7/1 -> position_to_speed_pll/4(ki_pll), Delay24/1
  Switch8/1 -> Goto8/1, Delay27/1
  Switch9/1 -> position_to_speed_pll/1(position_mech_SI)
  position_to_speed_pll/1(speed_mech_SI) -> Goto12/1
  slice_position_and_status/1(pos_raw_st) -> Gray_code_to_binary/1(ssi_pos_raw_single_turn)
  slice_position_and_status/2(pos_raw_mt) -> Gray_code_to_binary/3(ssi_pos_raw_multi_turn)
  slice_position_and_status/3(raw_status) -> Goto20/1
  ssi_communication/1(ssi_clk) -> Goto24/1
  ssi_communication/2(ssi_clk_enb_out) -> Goto6/1
  ssi_communication/3(ssi_clk_idle_levels) -> Goto23/1
  ssi_communication/4(ssi_data_raw) -> Goto21/1
  ssi_communication/5(ssi_data_out) -> Goto19/1
  ssi_communication/6(ssi_transaction_done) -> Goto17/1
  wrap_2pi/1(output) -> Delay42/1, Delay40/1
  wrap_2pi_after_offset/1(output) -> Goto14/1
  Goto17/1 -> From8/1, From15/1, From/1
  Goto1/1 -> From1/1
  Goto8/1 -> From11/1
  Goto2/1 -> From19/1, From12/1
  Goto10/1 -> From13/1
  Goto12/1 -> From31/1, From3/1, From14/1
  Goto11/1 -> From32/1, From16/1
  Goto16/1 -> From17/1
  Goto21/1 -> From18/1
  Goto4/1 -> From2/1
  Goto13/1 -> From20/1
  Goto14/1 -> From22/1, From21/1
  Goto/1 -> From36/1, From23/1
  Goto15/1 -> From35/1, From24/1
  Goto9/1 -> From37/1, From25/1
  Goto18/1 -> From27/1
  Goto6/1 -> From28/1
  Goto19/1 -> From29/1
  Goto20/1 -> From30/1
  Goto22/1 -> From39/1, From38/1
  Goto7/1 -> From4/1
  Goto23/1 -> From40/1
  Goto24/1 -> From5/1
  Goto5/1 -> From6/1
  Goto3/1 -> From7/1
  From32/1 -> delayMatch/1
  Delay127/1 -> delayMatch1/1
  Delay4/1 -> delayMatch2/1
  Delay7/1 -> delayMatch3/1
  Delay129/1 -> delayMatch4/1
  Switch6/1 -> delayMatch5/1, Goto4/1, Delay16/1, Delay15/1
  Delay16/1 -> delayMatch6/1
  Switch16/1 -> delayMatch7/1, Delay51/1, Delay50/1
  Delay51/1 -> delayMatch8/1
  Switch19/1 -> delayMatch9/1, Delay55/1, Delay54/1
  Delay55/1 -> delayMatch10/1
  Delay17/1 -> delayMatch11/1
  Delay10/1 -> delayMatch12/1
  Delay11/1 -> delayMatch13/1
  Delay40/1 -> delayMatch14/1
  Delay42/1 -> delayMatch15/1
  Delay24/1 -> Switch7/3
  Delay31/1 -> Switch31/3
  Delay1/1 -> Switch1/3
  Delay44/1 -> Switch13/3
  Delay48/1 -> Switch15/3
  Delay14/1 -> Switch5/3
  Delay52/1 -> Switch18/3
  Delay46/1 -> Switch14/3
  Delay15/1 -> Switch6/3
  Delay50/1 -> Switch16/3
  Delay54/1 -> Switch19/3
  Delay8/1 -> Switch2/3
  Delay37/1 -> Switch12/3
  Delay35/1 -> Switch11/3
  Delay29/1 -> Switch10/3
  Delay27/1 -> Switch8/3
  Delay20/1 -> Switch3/3
  Delay22/1 -> Switch4/3

== system gm_uz_ssi_interface_2023a/uz_ssi_interface/Gray_code_to_binary ==
  ssi_pos_raw_single_turn : Inport  OutDataTypeStr=uint32  PortDimensions=1  SampleTime=1e-08
  pos_is_binary_or_gray : Inport  Port=2  OutDataTypeStr=boolean  PortDimensions=1  SampleTime=1e-08
  ssi_pos_raw_multi_turn : Inport  Port=3  OutDataTypeStr=uint32  PortDimensions=1  SampleTime=1e-08
  trigger : Inport  Port=4  OutDataTypeStr=boolean  PortDimensions=1  SampleTime=1e-08
  Delay{,1,5..6} (4 alike) : Delay  DelayLength=double(1)  InitialCondition=0  SampleTime=1e-08
  Delay2 : Delay  DelayLength=double(101)  InitialCondition=0  SampleTime=1e-08
  Delay3 : Delay  DelayLength=double(101)  InitialCondition=0  SampleTime=1e-08
  Switch : Switch  Criteria=u2 > Threshold  Threshold=double(0)  OutDataTypeStr=uint32  SampleTime=1e-08  SaturateOnIntegerOverflow=off  InputSameDT=off
  Switch1 : Switch  Criteria=u2 > Threshold  Threshold=double(0)  OutDataTypeStr=uint32  SampleTime=1e-08  SaturateOnIntegerOverflow=off  InputSameDT=off
  gray_to_bin_mt : Subsystem
  gray_to_bin_st : Subsystem
  ssi_pos_single_turn_binary : Outport  SampleTime=1e-08
  ssi_pos_multi_turn_binary : Outport  Port=2  SampleTime=1e-08
  wires:
  Delay/1 -> gray_to_bin_st/1(gray)
  Delay1/1 -> gray_to_bin_mt/1(gray)
  Delay2/1 -> Switch/3
  Delay3/1 -> Switch1/3
  Delay5/1 -> Switch1/1
  Delay6/1 -> Switch/1
  Switch/1 -> ssi_pos_single_turn_binary/1
  Switch1/1 -> ssi_pos_multi_turn_binary/1
  gray_to_bin_mt/1(binary_out) -> Delay5/1
  gray_to_bin_st/1(binary_out) -> Delay6/1
  ssi_pos_raw_single_turn/1 -> Delay2/1, Delay/1
  pos_is_binary_or_gray/1 -> Switch1/2, Switch/2
  ssi_pos_raw_multi_turn/1 -> Delay3/1, Delay1/1
  trigger/1 -> gray_to_bin_mt/2(enb), gray_to_bin_st/2(enb)
